simulink model "reaction_wheels_design_v04"  (R2015b)
settings: Solver=VariableStepAuto  StartTime=0.0  StopTime=stop_time  RelTol=1e-6
values from neighbouring files (symbols this model uses):
  A = [zeros(3,3) eye(3);zeros(3,6)]    [main_reaction_wheels_design_v04.m]
  B = [zeros(3,3);diag([1/I_x 1/I_y 1/I_z])]    [main_nonlinear_spacecraft_euler.m]    (also in main_reaction_wheels_design_v04.m)
  C = eye(6)    [main_reaction_wheels_design_v04.m]
  D = zeros(6,3)    [main_reaction_wheels_design_v04.m]
  k_d_matrix = diag([k_d_x k_d_y k_d_z])    [main_reaction_wheels_design_v04.m]
  k_p_matrix = diag([k_p_x k_p_y k_p_z])    [main_reaction_wheels_design_v04.m]
  x_0 = [phi_0 ... (first row only)    [main_nonlinear_spacecraft_euler.m]    (also in main_nonlinear_spacecraft_quaternion.m = [epsilon_0; main_reaction_wheels_design_v04.m)
settings Model: Creator=Krunal's PC  LastModifiedBy=Krunal's PC

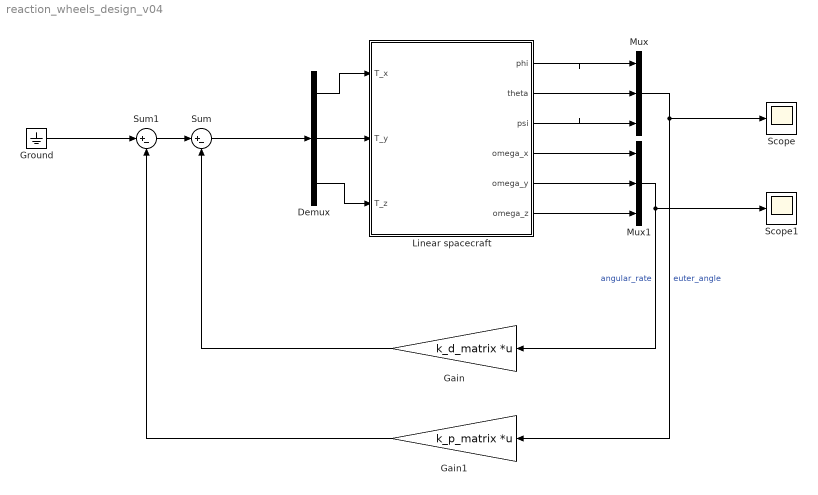
== system reaction_wheels_design_v04 ==
  Demux : Demux  Outputs=3
  Gain : Gain  Gain=k_d_matrix  Multiplication=Matrix(K*u)
  Gain1 : Gain  Gain=k_p_matrix  Multiplication=Matrix(K*u)
  Ground : Ground
  Linear spacecraft : Subsystem
  Mux : Mux  Inputs=3
  Mux1 : Mux  Inputs=3
  Scope : Scope
  Scope1 : Scope
  Sum : Sum  Inputs=|+-
  Sum1 : Sum  Inputs=|+-
  wires:
  Linear spacecraft/1(phi) -> Mux/1
  Linear spacecraft/2(theta) -> Mux/2
  Linear spacecraft/3(psi) -> Mux/3
  Linear spacecraft/4(omega_x) -> Mux1/1
  Linear spacecraft/5(omega_y) -> Mux1/2
  Linear spacecraft/6(omega_z) -> Mux1/3
  Mux1/1 -> Scope1/1, Gain/1  "angular_rate"
  Mux/1 -> Scope/1, Gain1/1  "euter_angle"
  Demux/1 -> Linear spacecraft/1(T_x)
  Demux/2 -> Linear spacecraft/2(T_y)
  Demux/3 -> Linear spacecraft/3(T_z)
  Gain/1 -> Sum/2
  Sum/1 -> Demux/1
  Sum1/1 -> Sum/1
  Gain1/1 -> Sum1/2
  Ground/1 -> Sum1/1

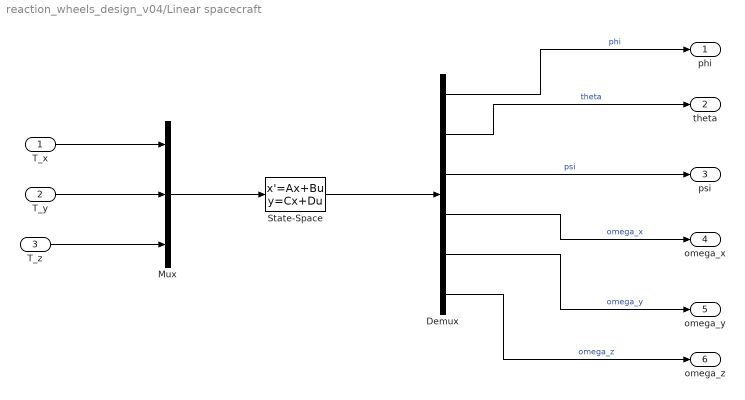
== system reaction_wheels_design_v04/Linear spacecraft ==
  T_x : Inport
  T_y : Inport  Port=2
  T_z : Inport  Port=3
  Demux : Demux  Outputs=6
  Mux : Mux  Inputs=3
  State-Space : StateSpace  A=A  B=B  C=C  D=D  X0=x_0
  phi : Outport
  theta : Outport  Port=2
  psi : Outport  Port=3
  omega_x : Outport  Port=4
  omega_y : Outport  Port=5
  omega_z : Outport  Port=6
  wires:
  T_z/1 -> Mux/3
  State-Space/1 -> Demux/1
  T_y/1 -> Mux/2
  Demux/2 -> theta/1  "theta"
  Demux/6 -> omega_z/1  "omega_z"
  T_x/1 -> Mux/1
  Mux/1 -> State-Space/1
  Demux/5 -> omega_y/1  "omega_y"
  Demux/3 -> psi/1  "psi"
  Demux/1 -> phi/1  "phi"
  Demux/4 -> omega_x/1  "omega_x"
